simulink model "Compensator_test"  (R2014a)
settings: Solver=ode45  StartTime=0.0  StopTime=1  FixedStep=dt/10  MaxStep=10*dt  MinStep=dt/1000  RelTol=1e-5
undefined symbols (not defined in the file or in its folder): amp_cl, Atf, Dtf
libraries: cstblocks x12
settings Model: Creator=Ron  LastModifiedBy=Ron
settings SolverCC: InitialStep=dt

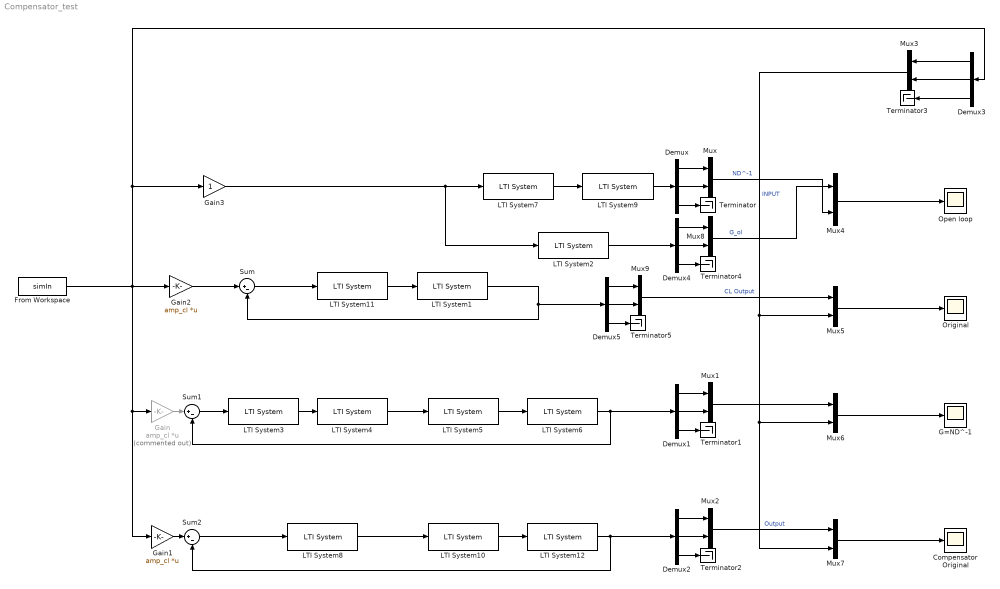
== system Compensator_test ==
  Compensator Original : Scope
      settings: ShowLegends=on  SaveName=ScopeData3
  Demux{,1..5} (6 alike) : Demux  Outputs=3
  From Workspace : FromWorkspace  VariableName=simIn  SampleTime=0
  G=ND^-1 : Scope
      settings: SaveName=ScopeData2
  Gain : Gain  Commented=on  Gain=amp_cl  Multiplication=Matrix(K*u)
  Gain1 : Gain  Gain=amp_cl  Multiplication=Matrix(K*u)
  Gain2 : Gain  Gain=amp_cl  Multiplication=Matrix(K*u)
  Gain3 : Gain
  LTI System1 : cstblocks/LTI System  sys=G_ol  IC=[0]
  LTI System10 : cstblocks/LTI System  sys=Ntf  IC=[0]
  LTI System11 : cstblocks/LTI System  sys=Ctf  IC=[0]
  LTI System12 : cstblocks/LTI System  sys=Dtf^-1  IC=[0]
  LTI System2 : cstblocks/LTI System  sys=G_ol  IC=[0]
  LTI System3 : cstblocks/LTI System  sys=Btf  IC=[0]
  LTI System4 : cstblocks/LTI System  sys=Atf^-1  IC=[0]
  LTI System5 : cstblocks/LTI System  sys=Dtf^-1  IC=[0]
  LTI System6 : cstblocks/LTI System  sys=Ntf  IC=[0]
  LTI System7 : cstblocks/LTI System  sys=Ntf  IC=[0]
  LTI System8 : cstblocks/LTI System  sys=Ctf  IC=[0]
  LTI System9 : cstblocks/LTI System  sys=Dtf^-1  IC=[0]
  Mux{,1..9} (10 alike) : Mux  Inputs=2
  Open loop : Scope
      settings: ShowLegends=on  YMin=-15  YMax=15
  Original : Scope
      settings: ShowLegends=on  YMin=-9e+54  YMax=-9676.64
  Sum : Sum  Inputs=|+-
  Sum1 : Sum  Inputs=|+-
  Sum2 : Sum  Inputs=|+-
  Terminator{,1..5} (6 alike) : Terminator
  wires:
  LTI System1/1 -> Sum/2, Demux5/1
  LTI System5/1 -> LTI System6/1
  Gain/1 -> Sum1/1
  Demux/1 -> Mux/1
  Demux/2 -> Mux/2
  Demux/3 -> Terminator/1
  Demux1/1 -> Mux1/1
  Demux1/2 -> Mux1/2
  Demux1/3 -> Terminator1/1
  LTI System6/1 -> Sum1/2, Demux1/1
  LTI System4/1 -> LTI System5/1
  LTI System3/1 -> LTI System4/1
  Sum1/1 -> LTI System3/1
  Sum/1 -> LTI System11/1
  LTI System11/1 -> LTI System1/1
  Demux3/2 -> Mux3/2
  Demux3/3 -> Terminator3/1
  Mux/1 -> Mux4/2  "ND^-1"
  Mux4/1 -> Open loop/1
  Demux3/1 -> Mux3/1
  Mux5/1 -> Original/1
  Mux1/1 -> Mux6/1
  Mux6/1 -> G=ND^-1/1
  LTI System10/1 -> LTI System12/1
  Gain1/1 -> Sum2/1
  Demux2/1 -> Mux2/1
  Demux2/2 -> Mux2/2
  Demux2/3 -> Terminator2/1
  LTI System12/1 -> Demux2/1, Sum2/2
  LTI System8/1 -> LTI System10/1
  Mux3/1 -> Mux7/2, Mux6/2, Mux5/2  "INPUT"
  Mux2/1 -> Mux7/1  "Output"
  Mux7/1 -> Compensator Original/1
  Sum2/1 -> LTI System8/1
  Gain2/1 -> Sum/1
  LTI System7/1 -> LTI System9/1
  From Workspace/1 -> Gain2/1, Gain3/1, Demux3/1, Gain1/1, Gain/1
  LTI System9/1 -> Demux/1
  Demux4/1 -> Mux8/1
  Demux4/2 -> Mux8/2
  Demux4/3 -> Terminator4/1
  LTI System2/1 -> Demux4/1
  Mux8/1 -> Mux4/1  "G_ol"
  Gain3/1 -> LTI System2/1, LTI System7/1
  Demux5/1 -> Mux9/1
  Demux5/2 -> Mux9/2
  Demux5/3 -> Terminator5/1
  Mux9/1 -> Mux5/1  "CL Output"
